simulink model "nldemo"  (R2020b)
settings: Solver=FixedStepAuto  StartTime=0.0  StopTime=inf  FixedStep=0.01  RelTol=1e-3
undefined symbols (not defined in the file): autopilot, control, kspTxIn0
libraries: ksplib x3
settings Model: DataDictionary=kspdemo.sldd  EnablePacing=on  PacingRate=2  Creator=brianhannan  LastModifiedBy=wizard

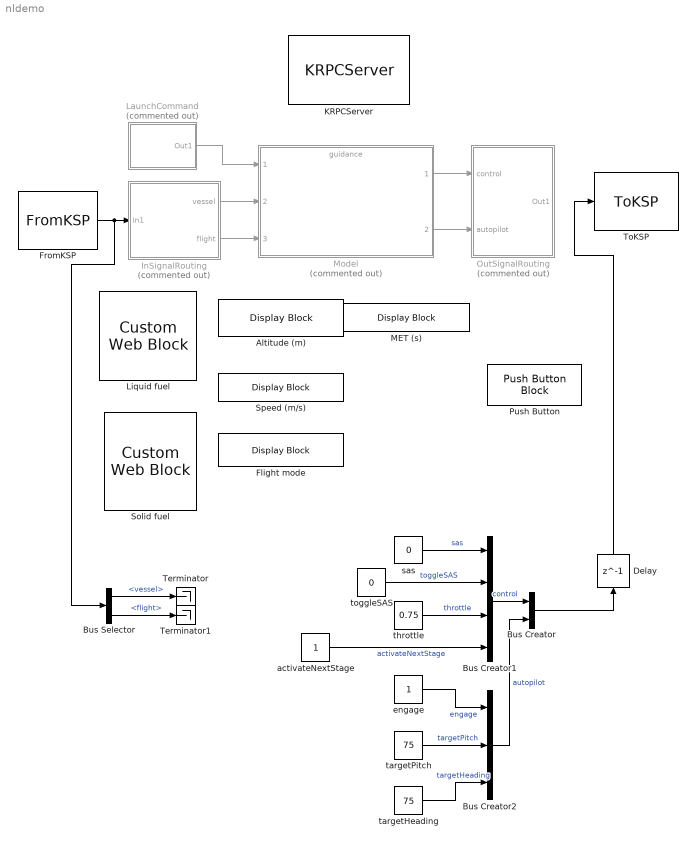
== system nldemo ==
  Altitude (m) : DisplayBlock  LabelPosition=Bottom  Format=short  Transparency=1
  Bus Creator : BusCreator  Inputs=2  OutDataTypeStr=Bus: kspTxIn  NonVirtualBus=on
  Bus Creator1 : BusCreator  Inputs=4  OutDataTypeStr=Bus: control  NonVirtualBus=on
  Bus Creator2 : BusCreator  Inputs=3  OutDataTypeStr=Bus: autopilot  NonVirtualBus=on
  Bus Selector : BusSelector  OutputSignals=vessel,flight
  Delay : Delay  DelayLength=1
  Flight mode : DisplayBlock  LabelPosition=Bottom  Format=short  Transparency=1
  FromKSP : ksplib/FromKSP
  InSignalRouting : Subsystem  Commented=on
  KRPCServer : ksplib/KRPCServer
  LaunchCommand : Subsystem  Commented=on  mask(Launch Command){launchCmd=logical(0)}
      mask prompts: launchCmd "Launch:"
      mask help: Send launch command
      mask Display: disp('Launch')
  Liquid fuel : CustomWebBlock  LabelPosition=Hide  ShowInitialText=on  Configuration="{\"components\":[{\"name\":\"CircularScaleComponent\",\"settings\":{\"bounds\":{\"max\":225,\"min\":0,\"tickInterval\":\"auto\"},\"direction\":\"cw\",\"flipLimits\":0,\"innerRadius\":0.75,\"internalTickHeightScaleFactor\":1,\"labelColor\":[255,252,199],\"labelFont\":{\"font\":\"Arial\",\"fontSize\":12},\"labelTransparency\":1,\"minorTickHeightScaleFactor\":0.2,\"needleImage\":{\"size\":[1890,567],\"src\":\"data:image\\/svg+xml;base64,PD94bWwgdmVyc2lvbj0iMS4wIiBlbmNvZGluZz0iVVRGLTgiIHN0YW5kYWxvbmU9Im5vIj8+CjxzdmcKICAgeG1sbnM6ZGM9Imh0dHA6Ly9wdXJsLm9yZy9kYy9lbGVtZW50cy8xLjEvIgogICB4bWxuczpjYz0iaHR0cDovL2NyZWF0aXZlY29tbW9ucy5vcmcvbnMjIgogICB4bWxuczpyZGY9Imh0dHA6Ly93d3cudzMub3JnLzE5OTkvMDIvMjItcmRmLXN5bnRheC1ucyMiCiAgIHhtbG5zOnN2Zz0iaHR0cDovL3d3dy53My5vcmcvMjAwMC9zdmciCiAgIHhtbG5zPSJodHRwOi8vd3d3LnczLm9yZy8yMDAwL3N2ZyIKICAgeG1sbnM6 ...(+4096 chars)\"},\"needleOffset\":[0.1610917094974375,0],\"needleOrientation\":-45,\"needleRotation\":180.59702388394928,\"needleSize\":{\"height\":0.13032601008944536,\"width\":0.416859542883425},\"outerRadius\":0.9,\"position\":[0.06486742424242424,0.05627705627705628,0.8917748917748918,0.8787878787878788],\"scaleAngle\":270,\"scaleAngleOffset\":135,\"scaleColors\":[],\"scaleColorsSize\":0.2,\"scalePosition\":[0,0,1,1],\"showLabels\":1,\"showMinorTicks\":1,\"showSpanLine\":1,\"showTicks\":1,\"tickColor\":[255,255,200],\"tickTransparency\":1,\"valueBarColor\":[0,114,189],\"valueBarPosition\":[0,0,1,1],\"valueBarSize\":0.2,\"valueBarTransparency\":1}},{\"name\":\"BackgroundImageComponent\",\"settings\":{\"image\":{\"size\":[500,500],\"src\":\"data:image\\/svg+xml;base64,PD94bWwgdmVyc2lvbj0iMS4wIiBlbmNvZGluZz0iVVRGLTgiIHN0YW5kYWxvbmU9Im5vIj8+CjxzdmcKICAgeG1sbnM6ZGM9Imh0dHA6Ly9wdXJsLm9yZy9kYy9lbGVtZW50cy8xLjEvIgogICB4bWxuczpjYz0iaHR0cDovL2NyZWF0aXZlY29tbW9ucy5vcmcvbnMjIgogICB4bWxuczpyZGY9Imh0dHA6Ly93d3cudzMub3JnLzE5OTkvMDIvMjItcmRmLXN5bnRheC1ucyMiCiAgIHhtbG5zOnN2Zz0iaHR0cDovL3d3dy53My5vcmcvMjAwMC9zdmciCiAgIHhtbG5zPSJodHRwOi8vd3d3LnczLm9yZy8yMDAwL3N2ZyIKICAgeG1sbnM6 ...(+9964 chars)\"},\"position\":[0,0,1,1],\"scaleMode\":\"0\"}},{\"name\":\"ForegroundImageComponent\",\"settings\":{\"image\":{\"size\":[0,0],\"src\":\"default\",\"srcOrientation\":[]},\"isForeground\":1,\"position\":[0,0,1,1],\"scaleMode\":\"0\"}}],\"settings\":{\"BindingType\":\"signal\",\"aspectRatio\":1.0318471337579618,\"direction\":\"cw\",\"fixedAspectRatio\":\"on\",\"flipLimits\":0,\"orientation\":\"horizontal\"},\"type\":\"CircularGauge\"}"
  MET (s) : DisplayBlock  LabelPosition=Bottom  Format=short  Transparency=1
  Model : ModelReference  Commented=on  ModelNameDialog=guidance  SimulationMode=Normal  ModelReferenceVersion=1.162
  OutSignalRouting : Subsystem  Commented=on
  Push Button : PushButtonBlock  ButtonText=Launch
  Solid fuel : CustomWebBlock  LabelPosition=Hide  ShowInitialText=on  Configuration="{\"components\":[{\"name\":\"CircularScaleComponent\",\"settings\":{\"bounds\":{\"max\":750,\"min\":0,\"tickInterval\":\"auto\"},\"direction\":\"cw\",\"flipLimits\":0,\"innerRadius\":0.75,\"internalTickHeightScaleFactor\":1,\"labelColor\":[255,252,199],\"labelFont\":{\"font\":\"Arial\",\"fontSize\":12},\"labelTransparency\":1,\"minorTickHeightScaleFactor\":0.2,\"needleImage\":{\"size\":[1890,567],\"src\":\"data:image\\/svg+xml;base64,PD94bWwgdmVyc2lvbj0iMS4wIiBlbmNvZGluZz0iVVRGLTgiIHN0YW5kYWxvbmU9Im5vIj8+CjxzdmcKICAgeG1sbnM6ZGM9Imh0dHA6Ly9wdXJsLm9yZy9kYy9lbGVtZW50cy8xLjEvIgogICB4bWxuczpjYz0iaHR0cDovL2NyZWF0aXZlY29tbW9ucy5vcmcvbnMjIgogICB4bWxuczpyZGY9Imh0dHA6Ly93d3cudzMub3JnLzE5OTkvMDIvMjItcmRmLXN5bnRheC1ucyMiCiAgIHhtbG5zOnN2Zz0iaHR0cDovL3d3dy53My5vcmcvMjAwMC9zdmciCiAgIHhtbG5zPSJodHRwOi8vd3d3LnczLm9yZy8yMDAwL3N2ZyIKICAgeG1sbnM6 ...(+4096 chars)\"},\"needleOffset\":[0.1610917094974375,0],\"needleOrientation\":-45,\"needleRotation\":180.59702388394928,\"needleSize\":{\"height\":0.13032601008944536,\"width\":0.416859542883425},\"outerRadius\":0.9,\"position\":[0.06486742424242424,0.05627705627705628,0.8917748917748918,0.8787878787878788],\"scaleAngle\":270,\"scaleAngleOffset\":135,\"scaleColors\":[],\"scaleColorsSize\":0.2,\"scalePosition\":[0,0,1,1],\"showLabels\":1,\"showMinorTicks\":1,\"showSpanLine\":1,\"showTicks\":1,\"tickColor\":[255,255,200],\"tickTransparency\":1,\"valueBarColor\":[0,114,189],\"valueBarPosition\":[0,0,1,1],\"valueBarSize\":0.2,\"valueBarTransparency\":1}},{\"name\":\"BackgroundImageComponent\",\"settings\":{\"image\":{\"size\":[500,500],\"src\":\"data:image\\/svg+xml;base64,PD94bWwgdmVyc2lvbj0iMS4wIiBlbmNvZGluZz0iVVRGLTgiIHN0YW5kYWxvbmU9Im5vIj8+CjxzdmcKICAgeG1sbnM6ZGM9Imh0dHA6Ly9wdXJsLm9yZy9kYy9lbGVtZW50cy8xLjEvIgogICB4bWxuczpjYz0iaHR0cDovL2NyZWF0aXZlY29tbW9ucy5vcmcvbnMjIgogICB4bWxuczpyZGY9Imh0dHA6Ly93d3cudzMub3JnLzE5OTkvMDIvMjItcmRmLXN5bnRheC1ucyMiCiAgIHhtbG5zOnN2Zz0iaHR0cDovL3d3dy53My5vcmcvMjAwMC9zdmciCiAgIHhtbG5zPSJodHRwOi8vd3d3LnczLm9yZy8yMDAwL3N2ZyIKICAgeG1sbnM6 ...(+9964 chars)\"},\"position\":[0,0,1,1],\"scaleMode\":\"0\"}},{\"name\":\"ForegroundImageComponent\",\"settings\":{\"image\":{\"size\":[0,0],\"src\":\"default\",\"srcOrientation\":[]},\"isForeground\":1,\"position\":[0,0,1,1],\"scaleMode\":\"0\"}}],\"settings\":{\"BindingType\":\"signal\",\"aspectRatio\":1.0318471337579618,\"direction\":\"cw\",\"fixedAspectRatio\":\"on\",\"flipLimits\":0,\"orientation\":\"horizontal\"},\"type\":\"CircularGauge\"}"
  Speed (m/s) : DisplayBlock  LabelPosition=Bottom  Format=short  Transparency=1
  Terminator : Terminator
  Terminator1 : Terminator
  ToKSP : ksplib/ToKSP
  activateNextStage : Constant  OutDataTypeStr=boolean
  engage : Constant  OutDataTypeStr=boolean
  sas : Constant  Value=0  OutDataTypeStr=boolean
  targetHeading : Constant  Value=75
  targetPitch : Constant  Value=75
  throttle : Constant  Value=0.75
  toggleSAS : Constant  Value=0  OutDataTypeStr=boolean
  wires:
  LaunchCommand/1(Out1) -> Model/1
  Model/1 -> OutSignalRouting/1(control)
  Model/2 -> OutSignalRouting/2(autopilot)
  Bus Creator/1 -> Delay/1
  FromKSP/1 -> InSignalRouting/1(In1), Bus Selector/1
  InSignalRouting/1(vessel) -> Model/2
  InSignalRouting/2(flight) -> Model/3
  Bus Selector/2 -> Terminator1/1  "<flight>"
  Bus Selector/1 -> Terminator/1  "<vessel>"
  throttle/1 -> Bus Creator1/3  "throttle"
  engage/1 -> Bus Creator2/1  "engage"
  targetPitch/1 -> Bus Creator2/2  "targetPitch"
  targetHeading/1 -> Bus Creator2/3  "targetHeading"
  Bus Creator2/1 -> Bus Creator/2  "autopilot"
  Bus Creator1/1 -> Bus Creator/1  "control"
  sas/1 -> Bus Creator1/1  "sas"
  toggleSAS/1 -> Bus Creator1/2  "toggleSAS"
  activateNextStage/1 -> Bus Creator1/4  "activateNextStage"
  Delay/1 -> ToKSP/1

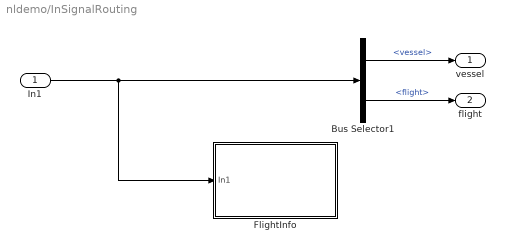
== system nldemo/InSignalRouting ==
  In1 : Inport
  Bus Selector1 : BusSelector  OutputSignals=vessel,flight
  FlightInfo : Subsystem
  vessel : Outport
  flight : Outport  Port=2
  wires:
  Bus Selector1/1 -> vessel/1  "<vessel>"
  Bus Selector1/2 -> flight/1  "<flight>"
  In1/1 -> FlightInfo/1(In1), Bus Selector1/1

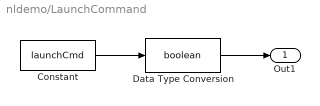
== system nldemo/LaunchCommand ==
  Constant : Constant  Value=launchCmd
  Data Type Conversion : DataTypeConversion  OutDataTypeStr=boolean
  Out1 : Outport
  wires:
  Constant/1 -> Data Type Conversion/1
  Data Type Conversion/1 -> Out1/1

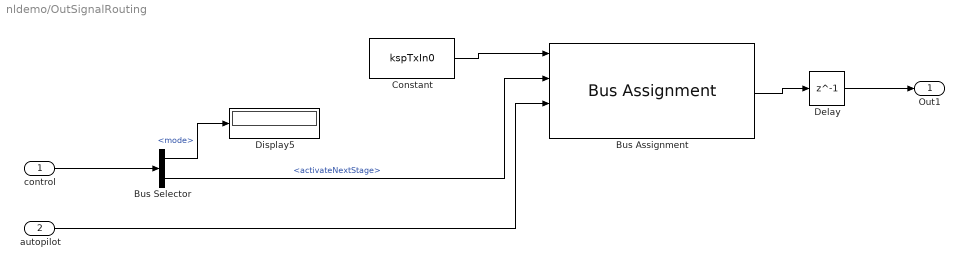
== system nldemo/OutSignalRouting ==
  control : Inport  OutDataTypeStr=Bus: mcout
  autopilot : Inport  Port=2  OutDataTypeStr=Bus: autopilot
  Bus Assignment : BusAssignment  AssignedSignals=control.activateNextStage,autopilot,control.throttle
  Bus Selector : BusSelector  OutputSignals=mode,activateNextStage
  Constant : Constant  Value=kspTxIn0  OutDataTypeStr=Bus: kspTxIn
  Delay : Delay  DelayLength=1
  Display5 : Display
  Out1 : Outport
  wires:
  Bus Assignment/1 -> Delay/1
  autopilot/1 -> Bus Assignment/3
  control/1 -> Bus Selector/1
  Bus Selector/2 -> Bus Assignment/2  "<activateNextStage>"
  Constant/1 -> Bus Assignment/1
  Bus Selector/1 -> Display5/1  "<mode>"
  Delay/1 -> Out1/1

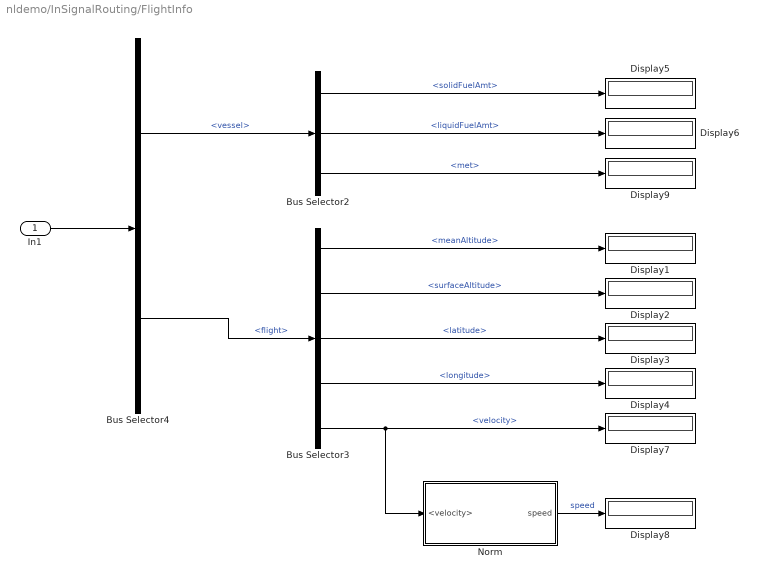
== system nldemo/InSignalRouting/FlightInfo ==
  In1 : Inport
  Bus Selector2 : BusSelector  OutputSignals=solidFuelAmt,liquidFuelAmt,met
  Bus Selector3 : BusSelector  OutputSignals=meanAltitude,surfaceAltitude,latitude,longitude,velocity
  Bus Selector4 : BusSelector  OutputSignals=vessel,flight
  Display{1..9} (9 alike) : Display
  Norm : Subsystem
  wires:
  Bus Selector2/2 -> Display6/1  "<liquidFuelAmt>"
  In1/1 -> Bus Selector4/1
  Bus Selector3/2 -> Display2/1  "<surfaceAltitude>"
  Bus Selector4/2 -> Bus Selector3/1  "<flight>"
  Bus Selector4/1 -> Bus Selector2/1  "<vessel>"
  Bus Selector3/4 -> Display4/1  "<longitude>"
  Bus Selector3/3 -> Display3/1  "<latitude>"
  Bus Selector3/1 -> Display1/1  "<meanAltitude>"
  Bus Selector2/1 -> Display5/1  "<solidFuelAmt>"
  Bus Selector3/5 -> Norm/1(<velocity>), Display7/1  "<velocity>"
  Norm/1(speed) -> Display8/1  "speed"
  Bus Selector2/3 -> Display9/1  "<met>"

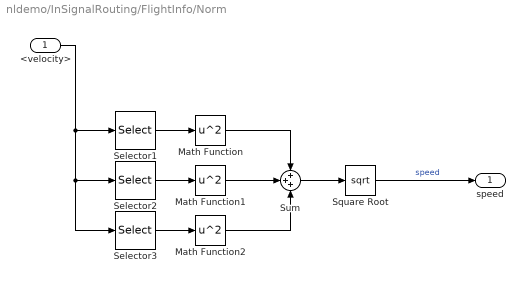
== system nldemo/InSignalRouting/FlightInfo/Norm ==
  <velocity> : Inport
  Math Function : Math  Operator=square  SaturateOnIntegerOverflow=on
  Math Function1 : Math  Operator=square  SaturateOnIntegerOverflow=on
  Math Function2 : Math  Operator=square  SaturateOnIntegerOverflow=on
  Selector1 : Selector  InputPortWidth=3  IndexOptions=Index vector (dialog)  Indices=1  OutputSizes=1
  Selector2 : Selector  InputPortWidth=3  IndexOptions=Index vector (dialog)  Indices=2  OutputSizes=1
  Selector3 : Selector  InputPortWidth=3  IndexOptions=Index vector (dialog)  Indices=3  OutputSizes=1
  Square Root : Sqrt  SaturateOnIntegerOverflow=on
  Sum : Sum  Inputs=+++
  speed : Outport
  wires:
  Square Root/1 -> speed/1  "speed"
  Selector1/1 -> Math Function/1
  Sum/1 -> Square Root/1
  Math Function2/1 -> Sum/3
  Math Function/1 -> Sum/1
  Math Function1/1 -> Sum/2
  Selector2/1 -> Math Function1/1
  Selector3/1 -> Math Function2/1
  <velocity>/1 -> Selector3/1, Selector2/1, Selector1/1
